simulink model "main_mb"  (Simulink 10.0)
settings: Solver=ode45  StartTime=0.0  StopTime=75001  RelTol=1e-3  EnableMultiTasking=on
libraries: simulink x1, powerlib x1
settings Model: Creator=giovanni  LastModifiedBy=marcomussi
settings DataIOCC: LimitDataPoints=on  SignalLoggingSaveFormat=ModelDataLogs
settings OptimizationCC: ExpressionDepthLimit=2147483647
settings DebuggingCC: SolverPrmCheckMsg=warning  FcnCallInpInsideContextMsg=warning  StateNameClashWarn=warning
settings GRTTargetCC: GeneratePreprocessorConditionals=Disable all
settings ConfigComp: CovExternalEMLEnable=off  CovSFcnEnable=off

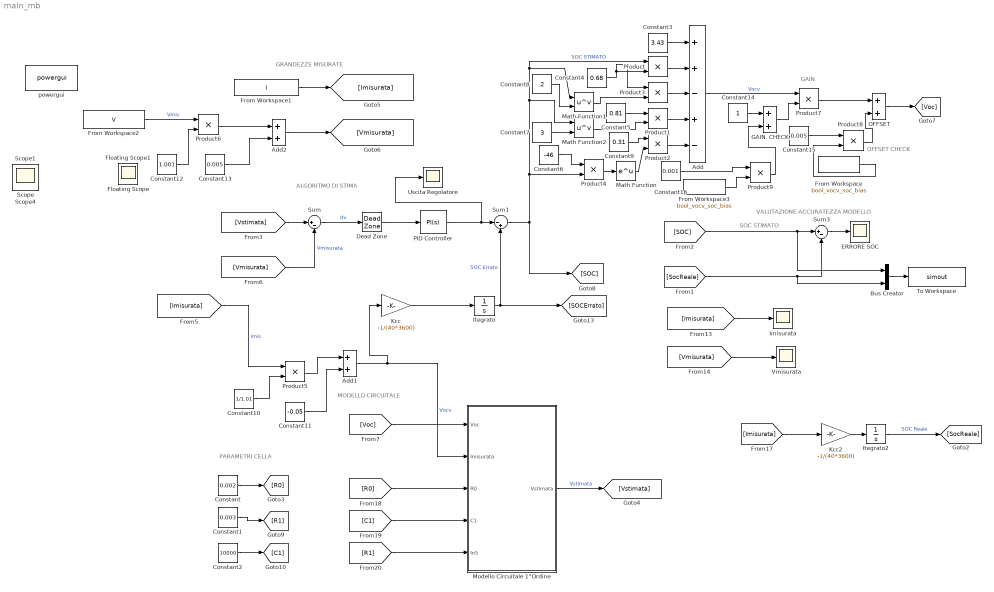
== system main_mb ==
  note: OFFSET
      | CHECK
  note: GAIN
  note: GRANDEZZE MISURATE
  note: PARAMETRI CELLA
  note: ALGORITMO DI STIMA
  note: MODELLO CIRCUITALE
  note: SOC STIMATO
  note: VALUTAZIONE ACCURATEZZA MODELLO
  Add : Sum  Inputs=++-+-
  Add1 : Sum
  Add2 : Sum
  Bus Creator : BusCreator  Inputs=2
  Constant : Constant  Value=0.002
  Constant1 : Constant  Value=0.003
  Constant10 : Constant  Value=1/1.01
  Constant11 : Constant  Value=-0.05
  Constant12 : Constant  Value=1.001
  Constant13 : Constant  Value=0.005
  Constant14 : Constant
  Constant15 : Constant  Value=0.005
  Constant16 : Constant  Value=0.001
  Constant2 : Constant  Value=10000
  Constant3 : Constant  Value=3.43
  Constant4 : Constant  Value=0.68
  Constant5 : Constant  Value=0.81
  Constant6 : Constant  Value=-46
  Constant7 : Constant  Value=3
  Constant8 : Constant  Value=2
  Constant9 : Constant  Value=0.31
  Dead Zone : DeadZone  LowerValue=-0.01  UpperValue=0.01  SaturateOnIntegerOverflow=on
  ERRORE SOC : Scope
  From Workspace : FromWorkspace  VariableName=bool_vocv_soc_bias  SampleTime=0
  From Workspace1 : FromWorkspace  VariableName=I  SampleTime=1
  From Workspace2 : FromWorkspace  VariableName=V  SampleTime=1
  From Workspace3 : FromWorkspace  VariableName=bool_vocv_soc_bias  SampleTime=0
  GAIN  CHECK : Sum
  Imisurata : Scope
  Itegrato : Integrator  InitialCondition=0.55
  Itegrato2 : Integrator  InitialCondition=0.55
  Kcc : Gain  Gain=-1/(40*3600)
  Kcc2 : Gain  Gain=-1/(40*3600)
  Math Function : Math  SignedPower=off  SaturateOnIntegerOverflow=on
  Math Function1 : Math  Operator=pow  SignedPower=off  SaturateOnIntegerOverflow=on
  Math Function2 : Math  Operator=pow  SignedPower=off  SaturateOnIntegerOverflow=on
  Modello Circuitale 1°Ordine : Subsystem
  OFFSET : Sum
  PID Controller : simulink/Continuous/PID Controller  Controller=PI  Form=Parallel  TimeDomain=Continuous-time  SampleTime=1  IntegratorMethod=Forward Euler  FilterMethod=Forward Euler  ControllerParametersSource=internal  P=0  I=0.01  D=0  UseFilter=on  N=100  TunerSelectOption=Transfer Function Based (PID Tuner App)  InitialConditionSource=internal  InitialConditionForIntegrator=0  InitialConditionForFilter=0  DifferentiatorICPrevScaledInput=0  ExternalReset=none  TrackingMode=off  Kt=1  LimitOutput=off  UpperSaturationLimit=inf  LowerSaturationLimit=-inf  LinearizeAsGain=off  AntiWindupMode=none  Kb=1  POutMin=[]  POutMax=[]  IOutMin=[]  IOutMax=[]  DOutMin=[]  DOutMax=[]  NOutMin=[]  NOutMax=[]  SumOutMin=[]  SumOutMax=[]  SaturationOutMin=[]  SaturationOutMax=[]  PParamMin=[]  PParamMax=[]  IParamMin=[]  IParamMax=[]  DParamMin=[]  DParamMax=[]  NParamMin=[]  NParamMax=[]  KbParamMin=[]  KbParamMax=[]  KtParamMin=[]  KtParamMax=[]  KbOutMin=[]  KbOutMax=[]  KtOutMin=[]  KtOutMax=[]  IntegratorOutMin=[]  IntegratorOutMax=[]  FilterOutMin=[]  FilterOutMax=[]  SumI1OutMin=[]  SumI1OutMax=[]  SumI2OutMin=[]  SumI2OutMax=[]  SumI3OutMin=[]  SumI3OutMax=[]  SumI4OutMin=[]  SumI4OutMax=[]  SumDOutMin=[]  SumDOutMax=[]  DifferentiatorOutMin=[]  DifferentiatorOutMax=[]  FilterDiffOutCoefMin=[]  FilterDiffOutCoefMax=[]  ReciprocalOutMin=[]  ReciprocalOutMax=[]  SumDenOutMin=[]  SumDenOutMax=[]  SumNumOutMin=[]  SumNumOutMax=[]  DivideOutMin=[]  DivideOutMax=[]  IntegratorContinuousStateAttributes=''  IntegratorStateMustResolveToSignalObject=off  IntegratorRTWStateStorageClass=Auto  FilterContinuousStateAttributes=''  FilterStateMustResolveToSignalObject=off  FilterRTWStateStorageClass=Auto  ParallelPVariant=InternalParameters  IdealPVariant=Disabled  IVariant=InternalParameters  DVariant=Disabled  IntegratorVariant=Continuous  SatVariant=Disabled  AWVariant=Passthrough  PCopyVariant=Disabled  TRVariant=Disabled  FdbkBlocksVariant=Forward  IdealPFdbkVariant=Disabled  SatFdbkVariant=Disabled  DerivativeFilterVariant=Disabled  NVariant=Disabled  NCopyVariant=Disabled_SignalSpec  FilterICVariant=Disabled  IntegratorICVariant=InternalICs  ExternalResetVariant=Disabled  TRSumVariant=Passthrough  SumFdbkVariant=Disabled  SumVariant=Sum_PI
      link override Integral Gain: Gain=I  Multiplication=Element-wise(K.*u)  ParamMin=IParamMin  ParamMax=IParamMax  ParamDataTypeStr=IParamDataTypeStr  OutMin=IOutMin  OutMax=IOutMax  OutDataTypeStr=IOutDataTypeStr  SampleTime=-1
  Product{,1..9} (10 alike) : Product
  Sum : Sum  Inputs=|+-
  Sum1 : Sum  Inputs=|-+
  Sum3 : Sum  Inputs=|+-
  To Workspace : ToWorkspace  VariableName=simout  SaveFormat=Timeseries  SampleTime=-1
  Uscita Regolatore : Scope
  Vmisurata : Scope
  powergui : powerlib/powergui  Priority=1  SimulationMode=Discrete  SampleTime=1  frequency=60  Iterations=50  frequencyindice=0  Pbase=100e6  ErrMax=1e-4  UnitsV=kV  UnitsW=MW  buscounter=0  FunctionMessages=off  echomessages=off  EnableUseOfTLC=off  CurrentSourceSwitches=off  DisableSnubberDevices=off  DisableRonSwitches=off  DisableVfSwitches=off  DisplayEquations=off  AutomaticDiscreteSolvers=off  SolverType=Tustin/Backward Euler (TBE)  Interpol=off  ExternalGateDelay=off  methode=off  Ts=100  x0status=blocks  SPID=on  SwTol=0  HookPort=off  NonlinearTolerance=1e-4  nMaxIteration=100  ContinueOnMaxIteration=off  RestoreLinks=warning  ResistiveCurrentMeasurement=off  Frange=[0:2:500]  Ylog=off  Xlog=on  ShowGrid=off  save=off  variable=ZData  structure=0  ZoomFFT=off  StartTime=0.0  cycles=1  DisplayStyle=1  fundamental=60  FreqAxis=off  MaxFrequency=1000  frequencyindicesteady=1  RmsSteady=1  display=off
      settings: SourceProductName=Simscape Electrical
  Floating Scope : Scope
  Floating Scope1 : Scope
  Scope : Scope
  Scope1 : Scope
  Scope4 : Scope
  wires:
  From Workspace1/1 -> [Imisurata]
  [Voc] -> Modello Circuitale 1°Ordine/1(Voc)
  [R1] -> Modello Circuitale 1°Ordine/5(In5)
  [R0] -> Modello Circuitale 1°Ordine/3(R0)
  [C1] -> Modello Circuitale 1°Ordine/4(C1)
  Sum1/1 -> Product4/2, Math Function2/1, Product/1, Math Function1/1, [SOC]  "SOC STIMATO"
  Kcc/1 -> Itegrato/1
  Itegrato/1 -> Sum1/2, [SOCErrato]  "SOC Errato"
  [Imisurata] -> Product5/1  "imis"
  [SOC] -> Bus Creator/1, Sum3/1
  Sum3/1 -> ERRORE SOC/1
  Modello Circuitale 1°Ordine/1(Vstimata) -> [Vstimata]  "Vstimata"
  [Imisurata] -> Imisurata/1
  [Vmisurata] -> Vmisurata/1
  Kcc2/1 -> Itegrato2/1
  [SocReale] -> Bus Creator/2, Sum3/2
  [Vstimata] -> Sum/1
  [Vmisurata] -> Sum/2  "Vmisurata"
  PID Controller/1 -> Sum1/1, Uscita Regolatore/1
  Sum/1 -> Dead Zone/1  "dv"
  Itegrato2/1 -> [SocReale]  "SOC Reale"
  Dead Zone/1 -> PID Controller/1
  Constant2/1 -> [C1]
  Constant/1 -> [R0]
  Constant1/1 -> [R1]
  Constant6/1 -> Product4/1
  Math Function/1 -> Product2/2
  Constant3/1 -> Add/1
  Math Function2/1 -> Product1/2
  Math Function1/1 -> Product3/2
  Constant8/1 -> Math Function1/2
  Constant7/1 -> Math Function2/2
  Product4/1 -> Math Function/1
  Constant9/1 -> Product2/1
  Product2/1 -> Add/5
  Constant5/1 -> Product1/1
  Constant4/1 -> Product3/1, Product/2
  Product1/1 -> Add/4
  Product3/1 -> Add/3
  Product/1 -> Add/2
  Bus Creator/1 -> To Workspace/1
  [Imisurata] -> Kcc2/1
  Product5/1 -> Add1/1
  Constant11/1 -> Add1/2
  Constant10/1 -> Product5/2
  Add1/1 -> Kcc/1, Modello Circuitale 1°Ordine/2(Imisurata)  "Vocv"
  Add2/1 -> [Vmisurata]
  Constant13/1 -> Add2/2
  Product6/1 -> Add2/1
  From Workspace2/1 -> Product6/1  "Vmis"
  Constant12/1 -> Product6/2
  Product7/1 -> OFFSET/1
  Add/1 -> Product7/1  "Vocv"
  OFFSET/1 -> [Voc]
  Product8/1 -> OFFSET/2
  Constant15/1 -> Product8/1
  From Workspace/1 -> Product8/2
  GAIN  CHECK/1 -> Product7/2
  Constant14/1 -> GAIN  CHECK/1
  Constant16/1 -> Product9/1
  From Workspace3/1 -> Product9/2
  Product9/1 -> GAIN  CHECK/2

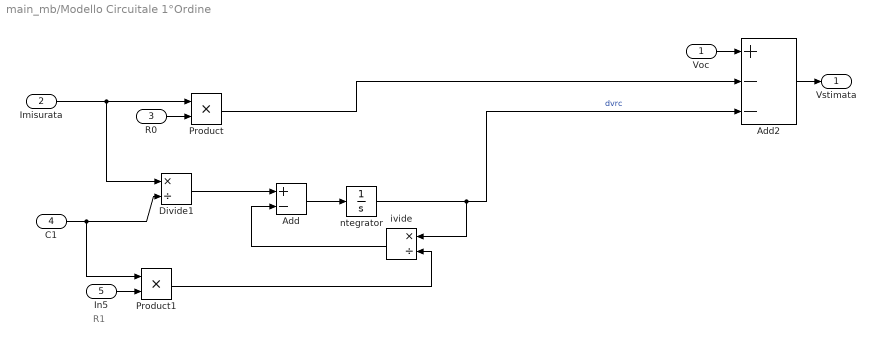
== system main_mb/Modello Circuitale 1°Ordine ==
  note: R1
  Voc : Inport
  Imisurata : Inport  Port=2
  R0 : Inport  Port=3
  C1 : Inport  Port=4
  In5 : Inport  Port=5
  Add : Sum  Inputs=+-
  Add2 : Sum  Inputs=+--
  Divide1 : Product  Inputs=*/
  Product : Product  RndMeth=Zero
  Product1 : Product  RndMeth=Zero
  ivide : Product  Inputs=*/
  ntegrator : Integrator
  Vstimata : Outport  VectorParamsAs1DForOutWhenUnconnected=off
  wires:
  Product/1 -> Add2/2
  ivide/1 -> Add/2
  Product1/1 -> ivide/2
  Divide1/1 -> Add/1
  C1/1 -> Divide1/2, Product1/1
  ntegrator/1 -> ivide/1, Add2/3  "dvrc"
  Add/1 -> ntegrator/1
  Imisurata/1 -> Product/1, Divide1/1
  Voc/1 -> Add2/1
  Add2/1 -> Vstimata/1
  R0/1 -> Product/2
  In5/1 -> Product1/2
